simulink model "sim_sfsp_Discreto"  (R2022a)
settings: Solver=VariableStepAuto  StartTime=0.0  StopTime=Tsim  MaxStep=0.01  RelTol=1e-3
values from neighbouring files (symbols this model uses):
  A_sin = 0.6    [SFSP_Discreto.m]
  A_step = 1e-2    (= 0.01)    [SFSP_Discreto.m]
  d = round(L/Ts)    [SFSP_Discreto.m]    (also in SFSPd.m = round(d/Ts))
  Freq = 1.35/(2*pi)    (= 0.214859173174)    [SFSP_Discreto.m]
  kr = eye(size(B,2))/(C/(eye(size(A)) + (-A + B*K))*B)    [SFSPd.m]
  ref = 1    [SFSP_Discreto.m]
  sd = 0    [SFSP_Discreto.m]
  t_step = 50    [SFSP_Discreto.m]
  Truido = 100    [SFSP_Discreto.m]
  Ts = 0.5    [SFSP_Discreto.m]
libraries: cstblocks x3, simulink x1
settings Model: Creator=Bismark  LastModifiedBy=Yo_Ju
settings SolverCC: AlgebraicLoopSolver=TrustRegion
settings DataIOCC: ReturnWorkspaceOutputs=off
settings DebuggingCC: UnconnectedInputMsg=warning  UnconnectedOutputMsg=warning  UnconnectedLineMsg=warning  SFMachineParentedDataDiag=warning  ArithmeticOperatorsInVariantConditions=warning
settings SFSimCC: SimUseLocalCustomCode=off  CustomCodeUndefinedFunction=UseInterfaceOnly
settings RTWCC: RTWUseLocalCustomCode=off
settings CodeAppCC: StateflowObjectComments=on

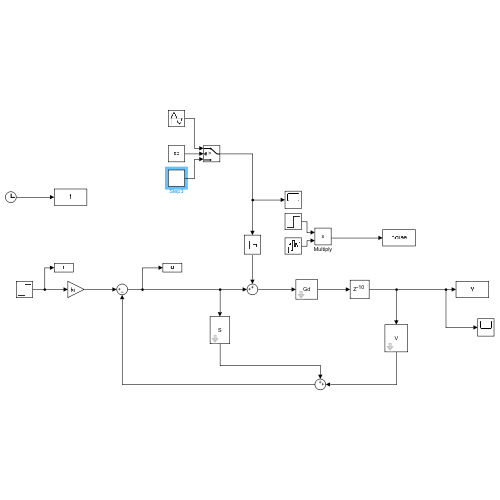
[thumbnail: Simulink's stored preview of the top-level diagram]
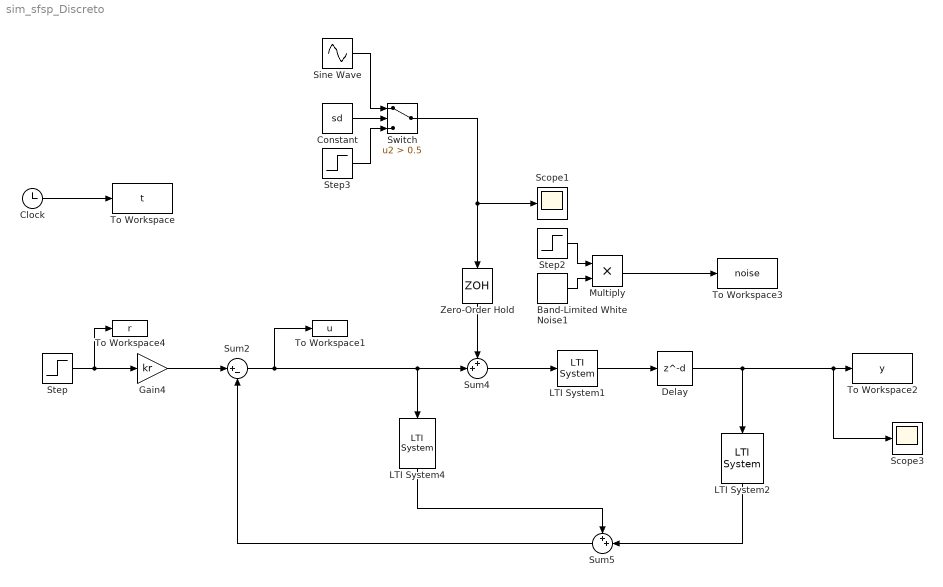
== system sim_sfsp_Discreto ==
  Band-Limited White Noise1 : simulink/Sources/Band-Limited White Noise  Cov=NoisePower  Ts=Ts  seed=[23341]
  Clock : Clock
  Constant : Constant  Value=sd
  Delay : Delay  DelayLength=d
  Gain4 : Gain  Gain=kr
  LTI System1 : cstblocks/LTI System  sys=Gd  IC=[]
  LTI System2 : cstblocks/LTI System  sys=V  IC=[]
  LTI System4 : cstblocks/LTI System  sys=S  IC=[]
  Multiply : Product
  Scope1 : Scope
  Scope3 : Scope
  Sine Wave : Sin  Amplitude=A_sin  Frequency=Freq  SampleTime=0
  Step : Step  Time=0  After=ref  SampleTime=0
  Step2 : Step  Time=Truido  SampleTime=0
  Step3 : Step  Time=t_step  After=A_step  SampleTime=0
  Sum2 : Sum  Inputs=|+-
  Sum4 : Sum  Inputs=++|
  Sum5 : Sum  Inputs=++|
  Switch : Switch  Criteria=u2 > Threshold  Threshold=0.5  SaturateOnIntegerOverflow=off  InputSameDT=off
  To Workspace : ToWorkspace  VariableName=t  SampleTime=Ts
  To Workspace1 : ToWorkspace  VariableName=u  SampleTime=Ts
  To Workspace2 : ToWorkspace  VariableName=y  SampleTime=Ts
  To Workspace3 : ToWorkspace  VariableName=noise  SampleTime=Ts
  To Workspace4 : ToWorkspace  VariableName=r  SampleTime=Ts
  Zero-Order Hold : ZeroOrderHold  SampleTime=Ts
  wires:
  Gain4/1 -> Sum2/1
  Clock/1 -> To Workspace/1
  Sum5/1 -> Sum2/2
  Delay/1 -> Scope3/1, To Workspace2/1, LTI System2/1
  LTI System2/1 -> Sum5/2
  Step/1 -> To Workspace4/1, Gain4/1
  LTI System4/1 -> Sum5/1
  Band-Limited White Noise1/1 -> Multiply/2
  Multiply/1 -> To Workspace3/1
  Step2/1 -> Multiply/1
  Sum4/1 -> LTI System1/1
  LTI System1/1 -> Delay/1
  Sum2/1 -> Sum4/2, LTI System4/1, To Workspace1/1
  Zero-Order Hold/1 -> Sum4/1
  Switch/1 -> Scope1/1, Zero-Order Hold/1
  Constant/1 -> Switch/2
  Sine Wave/1 -> Switch/1
  Step3/1 -> Switch/3
